simulink model "AttitudeTest"  (R2017b)
settings: Solver=ode45  StartTime=0.0  StopTime=20000  RelTol=1e-6  EnableMultiTasking=on
model workspace: external: MATLAB File C:\Users\Justin\Documents\00 MEng Project\PAN_ADCS\models\AttitudeTest_init.m (data not in the file)
undefined symbols (not defined in the file): accelmax, I, invI, Kd, Kp, muE, q_init, r_FWR, v_FWR, wbn_init, wmax, ww0
libraries: simulink x1
settings Model: Creator=Mason  LastModifiedBy=Justin
settings DataIOCC: LimitDataPoints=on  SaveFormat=Array  SignalLoggingSaveFormat=ModelDataLogs
settings OptimizationCC: ExpressionDepthLimit=2147483647  InitFltsAndDblsToZero=on  LifeSpan=inf
settings DebuggingCC: SaveWithParameterizedLinksMsg=none  UnderspecifiedInitializationDetection=Classic  MergeDetectMultiDrivingBlocksExec=none  SignalResolutionControl=TryResolveAllWithWarning  SolverPrmCheckMsg=warning  MultiTaskDSMMsg=warning  MultiTaskCondExecSysMsg=none  FcnCallInpInsideContextMsg=warning  StateNameClashWarn=warning  SFUnexpectedBacktrackingDiag=warning  SFNoUnconditionalDefaultTransitionDiag=warning  SFExecutionAtInitializationDiag=none
settings HardwareCC: ProdBitPerPointer=32  ProdBitPerSizeT=32  ProdBitPerPtrDiffT=32  ProdLargestAtomicFloat=None  ProdIntDivRoundTo=Undefined  ProdEndianess=Unspecified  ProdWordSize=32  ProdHWDeviceType=32-bit Generic
settings ModelReferenceCC: PropagateSignalLabelsOutOfModel=off
settings CodeAppCC: StateflowObjectComments=on
settings GRTTargetCC: TargetFcnLib=ansi_tfl_tmw.mat  TargetLangStandard=C89/C90 (ANSI)  GeneratePreprocessorConditionals=Disable all  CombineOutputUpdateFcns=off  GRTInterface=on
settings ConfigComp: CovMetricSettings=dw  CovHtmlReporting=on  CovSaveCumulativeToWorkspaceVar=on  CovSaveSingleToWorkspaceVar=on  CovExternalEMLEnable=off

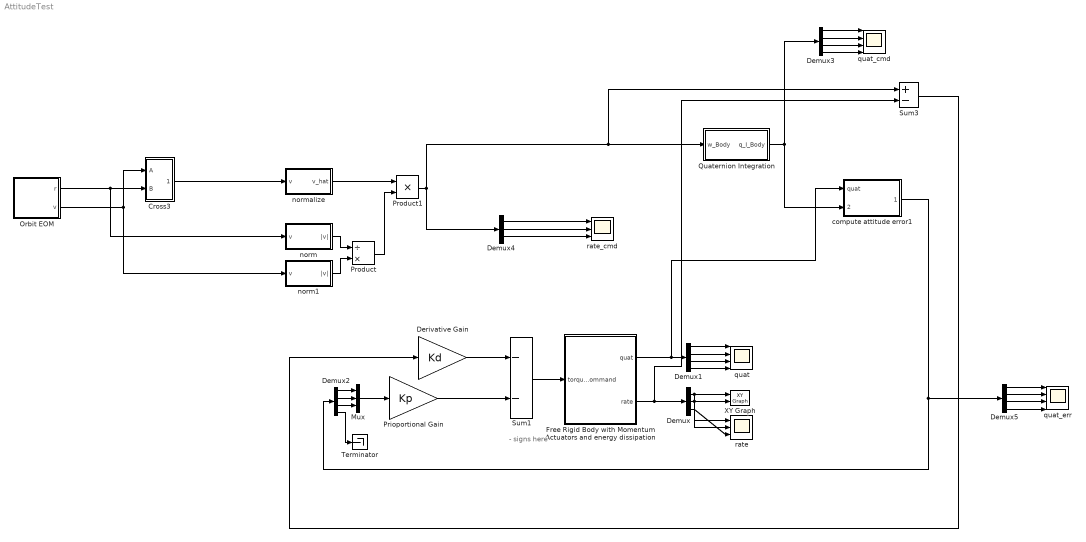
== system AttitudeTest ==
  note: - signs here
  Cross3 : Subsystem
  Demux : Demux  Outputs=3
  Demux{1..3,5} (4 alike) : Demux
  Demux4 : Demux  Outputs=3
  Derivative Gain : Gain  Gain=Kd  SaturateOnIntegerOverflow=on  OutDataTypeStr=Inherit: Same as input  ParamDataTypeStr=Inherit: Same as input
  Free Rigid Body with Momentum Actuators and energy dissipation : Subsystem
  Mux : Mux  Inputs=3
  Orbit EOM : Subsystem
  Prioportional Gain : Gain  Gain=Kp  SaturateOnIntegerOverflow=on  OutDataTypeStr=Inherit: Same as input  ParamDataTypeStr=Inherit: Same as input
  Product : Product  Inputs=/*
  Product1 : Product
  Quaternion Integration : Subsystem
  Sum1 : Sum  Inputs=--  SaturateOnIntegerOverflow=on  InputSameDT=on  OutDataTypeStr=Inherit: Same as first input
  Sum3 : Sum  Inputs=+-  SaturateOnIntegerOverflow=on  InputSameDT=on  OutDataTypeStr=Inherit: Same as first input
  Terminator : Terminator
  XY Graph : simulink/Sinks/XY Graph  xmin=-.1  xmax=.1  ymin=-.1  ymax=.1  st=.25
  compute attitude error1 : Subsystem
  norm : Subsystem
  norm1 : Subsystem
  normalize : Subsystem
  quat : Scope  NumInputPorts=4
  quat_cmd : Scope  NumInputPorts=4
  quat_err : Scope  NumInputPorts=4
  rate : Scope  NumInputPorts=3
  rate_cmd : Scope  NumInputPorts=3
  wires:
  Demux1/1 -> quat/1
  Demux1/2 -> quat/2
  Demux1/3 -> quat/3
  Demux1/4 -> quat/4
  Demux/1 -> rate/1, XY Graph/1
  Demux/2 -> rate/2, XY Graph/2
  Demux/3 -> rate/3
  Free Rigid Body with Momentum Actuators and energy dissipation/2(rate) -> Sum3/2, Demux/1
  Free Rigid Body with Momentum Actuators and energy dissipation/1(quat) -> compute attitude error1/1(quat), Demux1/1
  Sum1/1 -> Free Rigid Body with Momentum Actuators and energy dissipation/1(torque command)
  Mux/1 -> Prioportional Gain/1
  Derivative Gain/1 -> Sum1/1
  Demux2/2 -> Mux/2
  Demux2/1 -> Mux/1
  Demux2/3 -> Mux/3
  Demux2/4 -> Terminator/1
  Prioportional Gain/1 -> Sum1/2
  Quaternion Integration/1(q_I_Body) -> compute attitude error1/2(quat_cmd), Demux3/1
  compute attitude error1/1(quat error) -> Demux5/1, Demux2/1
  Sum3/1 -> Derivative Gain/1
  Product1/1 -> Demux4/1, Sum3/1, Quaternion Integration/1(w_Body)
  Demux3/3 -> quat_cmd/3
  Demux3/2 -> quat_cmd/2
  Demux3/4 -> quat_cmd/4
  Demux3/1 -> quat_cmd/1
  Orbit EOM/1(r) -> norm/1(v), Cross3/2(B)
  normalize/1(v_hat) -> Product1/1
  Product/1 -> Product1/2
  norm/1(|v|) -> Product/1
  Orbit EOM/2(v) -> Cross3/1(A), norm1/1(v)
  Cross3/1(AxB) -> normalize/1(v)
  norm1/1(|v|) -> Product/2
  Demux4/1 -> rate_cmd/1
  Demux4/3 -> rate_cmd/3
  Demux4/2 -> rate_cmd/2
  Demux5/2 -> quat_err/2
  Demux5/1 -> quat_err/1
  Demux5/4 -> quat_err/4
  Demux5/3 -> quat_err/3

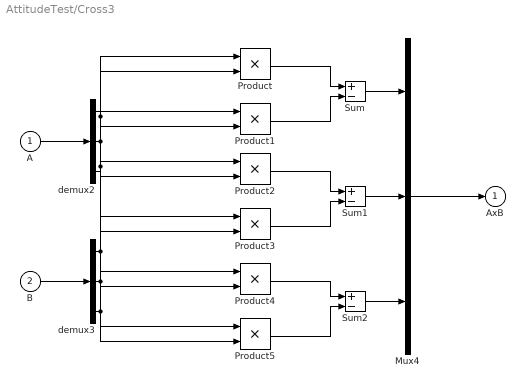
== system AttitudeTest/Cross3 ==
  A : Inport
  B : Inport  Port=2
  Mux4 : Mux  Inputs=3
  Product{,1..5} (6 alike) : Product  SaturateOnIntegerOverflow=on  InputSameDT=on  OutDataTypeStr=Inherit: Same as first input
  Sum : Sum  Inputs=+-  SaturateOnIntegerOverflow=on  InputSameDT=on  OutDataTypeStr=Inherit: Same as first input
  Sum1 : Sum  Inputs=+-  SaturateOnIntegerOverflow=on  InputSameDT=on  OutDataTypeStr=Inherit: Same as first input
  Sum2 : Sum  Inputs=+-  SaturateOnIntegerOverflow=on  InputSameDT=on  OutDataTypeStr=Inherit: Same as first input
  demux2 : Demux  Outputs=3
  demux3 : Demux  Outputs=3
  AxB : Outport  InitialOutput=0
  wires:
  A/1 -> demux2/1
  B/1 -> demux3/1
  demux2/3 -> Product1/1, Product2/1
  demux3/3 -> Product/2, Product3/2
  demux2/1 -> Product3/1, Product4/1
  demux3/2 -> Product1/2, Product4/2
  demux2/2 -> Product/1, Product5/1
  demux3/1 -> Product2/2, Product5/2
  Product/1 -> Sum/1
  Product1/1 -> Sum/2
  Product2/1 -> Sum1/1
  Product3/1 -> Sum1/2
  Product4/1 -> Sum2/1
  Product5/1 -> Sum2/2
  Sum/1 -> Mux4/1
  Sum1/1 -> Mux4/2
  Sum2/1 -> Mux4/3
  Mux4/1 -> AxB/1

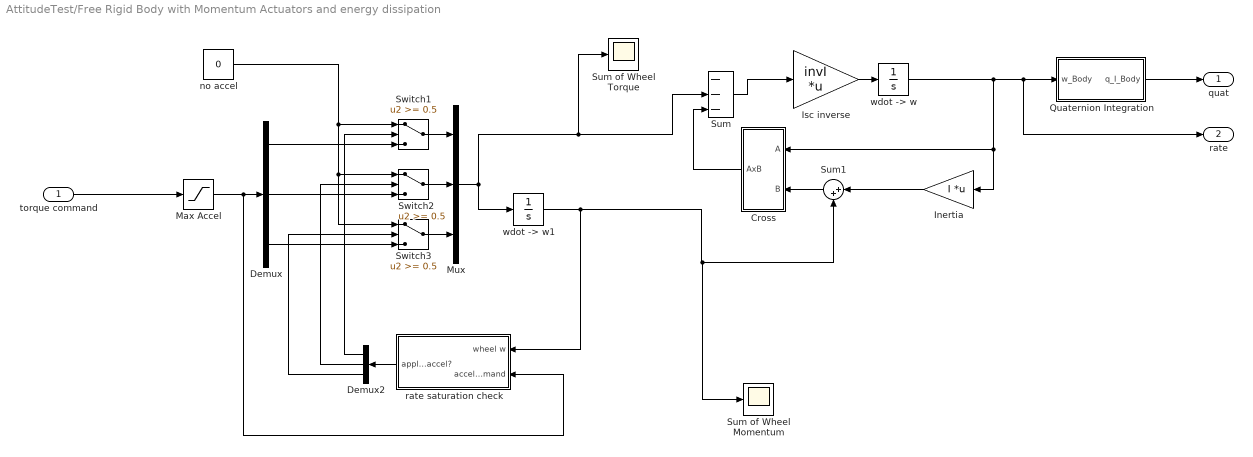
== system AttitudeTest/Free Rigid Body with Momentum Actuators and energy dissipation ==
  torque command : Inport
  Cross : Subsystem
  Demux : Demux  Outputs=3
  Demux2 : Demux  Outputs=3
  Inertia : Gain  Gain=I  Multiplication=Matrix(K*u)  SaturateOnIntegerOverflow=on  OutDataTypeStr=Inherit: Same as input  ParamDataTypeStr=Inherit: Same as input
  Isc inverse : Gain  Gain=invI  Multiplication=Matrix(K*u)  SaturateOnIntegerOverflow=on  OutDataTypeStr=Inherit: Same as input  ParamDataTypeStr=Inherit: Same as input
  Max Accel : Saturate  UpperLimit=accelmax  LowerLimit=-accelmax
  Mux : Mux  Inputs=3
  Quaternion Integration : Subsystem
  Sum : Sum  Inputs=|---  SaturateOnIntegerOverflow=on  InputSameDT=on  OutDataTypeStr=Inherit: Same as first input
  Sum of Wheel Momentum : Scope
  Sum of Wheel Torque : Scope
  Sum1 : Sum  Inputs=|++  SaturateOnIntegerOverflow=on  InputSameDT=on  OutDataTypeStr=Inherit: Same as first input
  Switch1 : Switch  Threshold=0.5  SaturateOnIntegerOverflow=on  InputSameDT=on
  Switch2 : Switch  Threshold=0.5  SaturateOnIntegerOverflow=on  InputSameDT=on
  Switch3 : Switch  Threshold=0.5  SaturateOnIntegerOverflow=on  InputSameDT=on
  no accel : Constant  Value=0
  rate saturation check : Subsystem
  "wdot -> w" : Integrator  InitialCondition=wbn_init
  "wdot -> w1" : Integrator  InitialCondition=ww0
  quat : Outport
  rate : Outport  Port=2
  wires:
  Isc inverse/1 -> "wdot -> w"/1
  "wdot -> w"/1 -> rate/1, Quaternion Integration/1(w_Body), Inertia/1, Cross/1(A)
  Sum/1 -> Isc inverse/1
  Cross/1(AxB) -> Sum/3
  Max Accel/1 -> rate saturation check/2(accel command), Demux/1
  Demux2/1 -> Switch1/2
  Demux2/2 -> Switch2/2
  Demux2/3 -> Switch3/2
  no accel/1 -> Switch1/1, Switch2/1, Switch3/1
  torque command/1 -> Max Accel/1
  Mux/1 -> Sum of Wheel Torque/1, Sum/2, "wdot -> w1"/1
  "wdot -> w1"/1 -> Sum of Wheel Momentum/1, Sum1/2, rate saturation check/1(wheel w)
  Inertia/1 -> Sum1/1
  Sum1/1 -> Cross/2(B)
  Quaternion Integration/1(q_I_Body) -> quat/1
  Switch1/1 -> Mux/1
  Switch2/1 -> Mux/2
  Switch3/1 -> Mux/3
  Demux/1 -> Switch1/3
  Demux/2 -> Switch2/3
  Demux/3 -> Switch3/3
  rate saturation check/1(apply accel?) -> Demux2/1

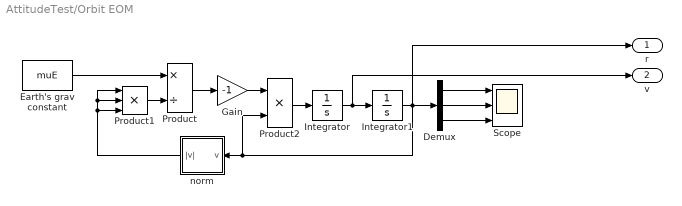
== system AttitudeTest/Orbit EOM ==
  Demux : Demux  Outputs=3
  Earth's grav constant : Constant  Value=muE
  Gain : Gain  Gain=-1  SaturateOnIntegerOverflow=on  OutDataTypeStr=Inherit: Same as input  ParamDataTypeStr=Inherit: Same as input
  Integrator : Integrator  InitialCondition=v_FWR
  Integrator1 : Integrator  InitialCondition=r_FWR
  Product : Product  Inputs=*/  SaturateOnIntegerOverflow=on  OutDataTypeStr=Inherit: Same as first input
  Product1 : Product  Inputs=***  SaturateOnIntegerOverflow=on  OutDataTypeStr=Inherit: Same as first input
  Product2 : Product  Inputs=**  SaturateOnIntegerOverflow=on  OutDataTypeStr=Inherit: Same as first input
  Scope : Scope  NumInputPorts=3
  norm : Subsystem
  r : Outport
  v : Outport  Port=2
  wires:
  norm/1(|v|) -> Product1/3, Product1/2, Product1/1
  Demux/3 -> Scope/3
  Demux/2 -> Scope/2
  Demux/1 -> Scope/1
  Gain/1 -> Product2/1
  Integrator/1 -> v/1, Integrator1/1
  Product2/1 -> Integrator/1
  Product/1 -> Gain/1
  Integrator1/1 -> r/1, Demux/1, norm/1(v), Product2/2
  Product1/1 -> Product/2
  Earth's grav constant/1 -> Product/1

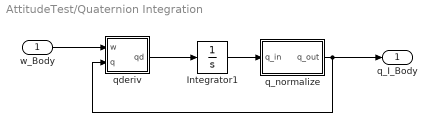
== system AttitudeTest/Quaternion Integration ==
  w_Body : Inport
  Integrator1 : Integrator  InitialCondition=q_init
  q_normalize : Subsystem
  qderiv : Subsystem
  q_I_Body : Outport
  wires:
  w_Body/1 -> qderiv/1(w)
  q_normalize/1(q_out) -> qderiv/2(q), q_I_Body/1
  Integrator1/1 -> q_normalize/1(q_in)
  qderiv/1(qd) -> Integrator1/1

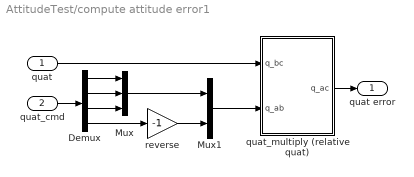
== system AttitudeTest/compute attitude error1 ==
  quat : Inport
  quat_cmd : Inport  Port=2
  Demux : Demux
  Mux : Mux  Inputs=3
  Mux1 : Mux  Inputs=2
  quat_multiply (relative quat) : Subsystem
  reverse : Gain  Gain=-1  SaturateOnIntegerOverflow=on  OutDataTypeStr=Inherit: Same as input  ParamDataTypeStr=Inherit: Same as input
  quat error : Outport
  wires:
  quat/1 -> quat_multiply (relative quat)/1(q_bc)
  quat_cmd/1 -> Demux/1
  Demux/1 -> Mux/1
  Demux/2 -> Mux/2
  Demux/3 -> Mux/3
  Demux/4 -> reverse/1
  Mux/1 -> Mux1/1
  Mux1/1 -> quat_multiply (relative quat)/2(q_ab)
  reverse/1 -> Mux1/2
  quat_multiply (relative quat)/1(q_ac) -> quat error/1

== system AttitudeTest/norm ==
  v : Inport
  Dot Product : DotProduct  InputSameDT=on  OutDataTypeStr=Inherit: Inherit via internal rule
  Math Function : Math  Operator=sqrt  SaturateOnIntegerOverflow=on
  |v| : Outport
  wires:
  Math Function/1 -> |v|/1
  Dot Product/1 -> Math Function/1
  v/1 -> Dot Product/2, Dot Product/1

== system AttitudeTest/norm1 ==
  v : Inport
  Dot Product : DotProduct  InputSameDT=on  OutDataTypeStr=Inherit: Inherit via internal rule
  Math Function : Math  Operator=sqrt  SaturateOnIntegerOverflow=on
  |v| : Outport
  wires:
  v/1 -> Dot Product/1, Dot Product/2
  Dot Product/1 -> Math Function/1
  Math Function/1 -> |v|/1

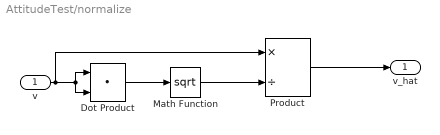
== system AttitudeTest/normalize ==
  v : Inport
  Dot Product : DotProduct  InputSameDT=on  OutDataTypeStr=Inherit: Inherit via internal rule
  Math Function : Math  Operator=sqrt  SaturateOnIntegerOverflow=on
  Product : Product  Inputs=*/  SaturateOnIntegerOverflow=on  InputSameDT=on  OutDataTypeStr=Inherit: Same as first input
  v_hat : Outport
  wires:
  v/1 -> Dot Product/1, Dot Product/2, Product/1
  Dot Product/1 -> Math Function/1
  Math Function/1 -> Product/2
  Product/1 -> v_hat/1

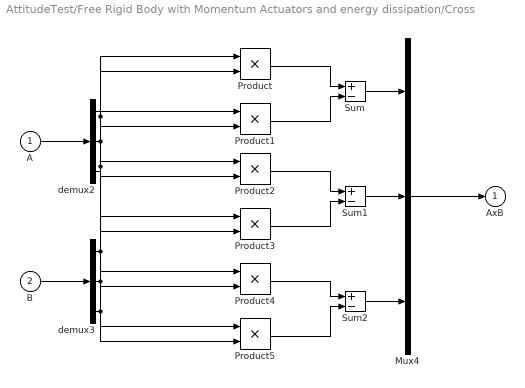
== system AttitudeTest/Free Rigid Body with Momentum Actuators and energy dissipation/Cross ==
  A : Inport
  B : Inport  Port=2
  Mux4 : Mux  Inputs=3
  Product{,1..5} (6 alike) : Product  SaturateOnIntegerOverflow=on  InputSameDT=on  OutDataTypeStr=Inherit: Same as first input
  Sum : Sum  Inputs=+-  SaturateOnIntegerOverflow=on  InputSameDT=on  OutDataTypeStr=Inherit: Same as first input
  Sum1 : Sum  Inputs=+-  SaturateOnIntegerOverflow=on  InputSameDT=on  OutDataTypeStr=Inherit: Same as first input
  Sum2 : Sum  Inputs=+-  SaturateOnIntegerOverflow=on  InputSameDT=on  OutDataTypeStr=Inherit: Same as first input
  demux2 : Demux  Outputs=3
  demux3 : Demux  Outputs=3
  AxB : Outport  InitialOutput=0
  wires:
  A/1 -> demux2/1
  B/1 -> demux3/1
  demux2/3 -> Product1/1, Product2/1
  demux3/3 -> Product/2, Product3/2
  demux2/1 -> Product3/1, Product4/1
  demux3/2 -> Product1/2, Product4/2
  demux2/2 -> Product/1, Product5/1
  demux3/1 -> Product2/2, Product5/2
  Product/1 -> Sum/1
  Product1/1 -> Sum/2
  Product2/1 -> Sum1/1
  Product3/1 -> Sum1/2
  Product4/1 -> Sum2/1
  Product5/1 -> Sum2/2
  Sum/1 -> Mux4/1
  Sum1/1 -> Mux4/2
  Sum2/1 -> Mux4/3
  Mux4/1 -> AxB/1

== system AttitudeTest/Free Rigid Body with Momentum Actuators and energy dissipation/Quaternion Integration ==
  w_Body : Inport
  Integrator1 : Integrator  InitialCondition=q_init
  q_normalize : Subsystem
  qderiv : Subsystem
  q_I_Body : Outport
  wires:
  w_Body/1 -> qderiv/1(w)
  q_normalize/1(q_out) -> qderiv/2(q), q_I_Body/1
  Integrator1/1 -> q_normalize/1(q_in)
  qderiv/1(qd) -> Integrator1/1

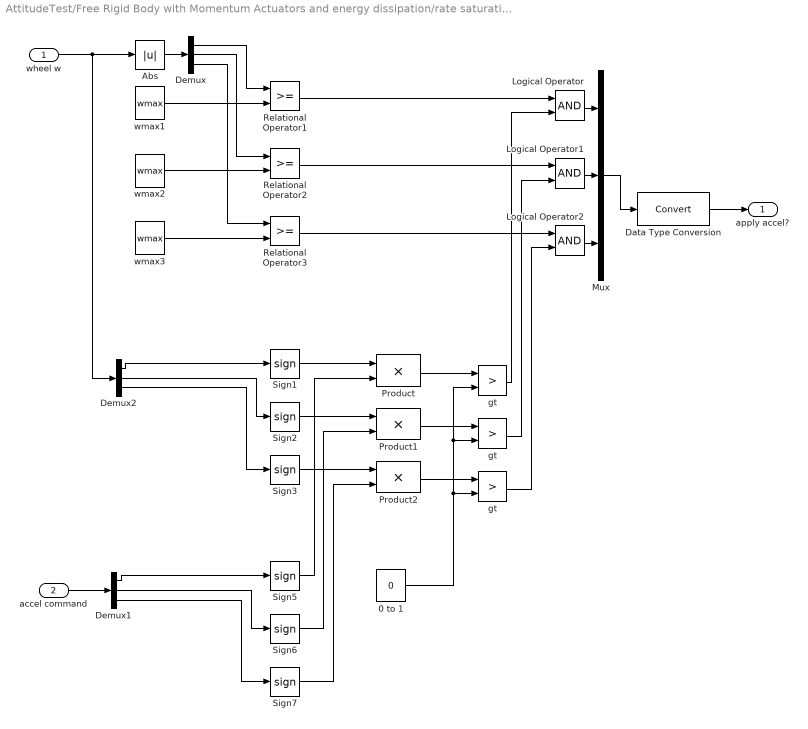
== system AttitudeTest/Free Rigid Body with Momentum Actuators and energy dissipation/rate saturation check ==
  wheel w : Inport
  accel command : Inport  Port=2
  0 to 1 : Constant  Value=0  VectorParams1D=off
  Abs : Abs  SaturateOnIntegerOverflow=on
  Data Type Conversion : DataTypeConversion
  Demux : Demux  Outputs=3
  Demux1 : Demux  Outputs=3
  Demux2 : Demux  Outputs=3
  Logical Operator : Logic
  Logical Operator1 : Logic
  Logical Operator2 : Logic
  Mux : Mux  Inputs=3
  Product : Product  SaturateOnIntegerOverflow=on  InputSameDT=on  OutDataTypeStr=Inherit: Same as first input
  Product1 : Product  SaturateOnIntegerOverflow=on  InputSameDT=on  OutDataTypeStr=Inherit: Same as first input
  Product2 : Product  SaturateOnIntegerOverflow=on  InputSameDT=on  OutDataTypeStr=Inherit: Same as first input
  Relational Operator1 : RelationalOperator  RndMeth=Nearest  InputSameDT=on
  Relational Operator2 : RelationalOperator  RndMeth=Nearest  InputSameDT=on
  Relational Operator3 : RelationalOperator  RndMeth=Nearest  InputSameDT=on
  Sign{1..3,5..7} (6 alike) : Signum
  gt : RelationalOperator  Operator=>  RndMeth=Nearest  InputSameDT=on
  "gt " : RelationalOperator  Operator=>  RndMeth=Nearest  InputSameDT=on
  "gt  " : RelationalOperator  Operator=>  RndMeth=Nearest  InputSameDT=on
  wmax1 : Constant  Value=wmax  VectorParams1D=off
  wmax2 : Constant  Value=wmax  VectorParams1D=off
  wmax3 : Constant  Value=wmax  VectorParams1D=off
  apply accel? : Outport
  wires:
  Abs/1 -> Demux/1
  Demux/1 -> Relational Operator1/1
  Demux/2 -> Relational Operator2/1
  Demux/3 -> Relational Operator3/1
  wmax1/1 -> Relational Operator1/2
  wmax2/1 -> Relational Operator2/2
  wmax3/1 -> Relational Operator3/2
  wheel w/1 -> Abs/1, Demux2/1
  Mux/1 -> Data Type Conversion/1
  accel command/1 -> Demux1/1
  Demux1/2 -> Sign6/1
  Demux1/3 -> Sign7/1
  Sign1/1 -> Product/1
  Sign5/1 -> Product/2
  Sign2/1 -> Product1/1
  Sign6/1 -> Product1/2
  Sign3/1 -> Product2/1
  Sign7/1 -> Product2/2
  Product/1 -> gt/1
  Product1/1 -> "gt "/1
  Product2/1 -> "gt  "/1
  Logical Operator/1 -> Mux/1
  Logical Operator1/1 -> Mux/2
  Logical Operator2/1 -> Mux/3
  Relational Operator1/1 -> Logical Operator/1
  Relational Operator2/1 -> Logical Operator1/1
  Relational Operator3/1 -> Logical Operator2/1
  gt/1 -> Logical Operator/2
  "gt "/1 -> Logical Operator1/2
  "gt  "/1 -> Logical Operator2/2
  Demux2/1 -> Sign1/1
  Demux2/2 -> Sign2/1
  Demux2/3 -> Sign3/1
  0 to 1/1 -> "gt  "/2, "gt "/2, gt/2
  Demux1/1 -> Sign5/1
  Data Type Conversion/1 -> apply accel?/1

== system AttitudeTest/Orbit EOM/norm ==
  v : Inport
  Dot Product : DotProduct  InputSameDT=on  OutDataTypeStr=Inherit: Inherit via internal rule
  Math Function : Math  Operator=sqrt  SaturateOnIntegerOverflow=on
  Saturation : Saturate  UpperLimit=1e20  LowerLimit=1e-10
  |v| : Outport
  wires:
  Saturation/1 -> |v|/1
  Math Function/1 -> Saturation/1
  Dot Product/1 -> Math Function/1
  v/1 -> Dot Product/2, Dot Product/1

== system AttitudeTest/Quaternion Integration/q_normalize ==
  q_in : Inport  PortDimensions=4
  Dot Product : DotProduct  InputSameDT=on  OutDataTypeStr=Inherit: Inherit via internal rule
  Math Function : Math  Operator=sqrt  SaturateOnIntegerOverflow=on
  Product : Product  Inputs=*/  SaturateOnIntegerOverflow=on  InputSameDT=on  OutDataTypeStr=Inherit: Same as first input
  q_out : Outport
  wires:
  Product/1 -> q_out/1
  Math Function/1 -> Product/2
  Dot Product/1 -> Math Function/1
  q_in/1 -> Product/1, Dot Product/2, Dot Product/1

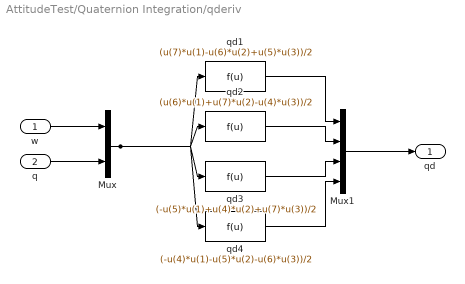
== system AttitudeTest/Quaternion Integration/qderiv ==
  w : Inport
  q : Inport  Port=2
  Mux : Mux  Inputs=2
  Mux1 : Mux
  qd1 : Fcn  Expr=(u(7)*u(1)-u(6)*u(2)+u(5)*u(3))/2
  qd2 : Fcn  Expr=(u(6)*u(1)+u(7)*u(2)-u(4)*u(3))/2
  qd3 : Fcn  Expr=(-u(5)*u(1)+u(4)*u(2)+u(7)*u(3))/2
  qd4 : Fcn  Expr=(-u(4)*u(1)-u(5)*u(2)-u(6)*u(3))/2
  qd : Outport
  wires:
  Mux1/1 -> qd/1
  qd4/1 -> Mux1/4
  qd3/1 -> Mux1/3
  qd2/1 -> Mux1/2
  qd1/1 -> Mux1/1
  Mux/1 -> qd4/1, qd3/1, qd2/1, qd1/1
  q/1 -> Mux/2
  w/1 -> Mux/1

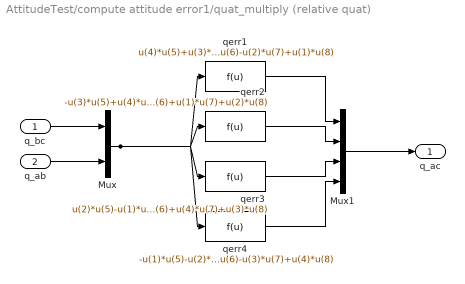
== system AttitudeTest/compute attitude error1/quat_multiply (relative quat) ==
  q_bc : Inport
  q_ab : Inport  Port=2
  Mux : Mux  Inputs=2
  Mux1 : Mux
  qerr1 : Fcn  Expr=u(4)*u(5)+u(3)*u(6)-u(2)*u(7)+u(1)*u(8)
  qerr2 : Fcn  Expr=-u(3)*u(5)+u(4)*u(6)+u(1)*u(7)+u(2)*u(8)
  qerr3 : Fcn  Expr=u(2)*u(5)-u(1)*u(6)+u(4)*u(7)+u(3)*u(8)
  qerr4 : Fcn  Expr=-u(1)*u(5)-u(2)*u(6)-u(3)*u(7)+u(4)*u(8)
  q_ac : Outport
  wires:
  Mux1/1 -> q_ac/1
  qerr4/1 -> Mux1/4
  qerr3/1 -> Mux1/3
  qerr2/1 -> Mux1/2
  qerr1/1 -> Mux1/1
  Mux/1 -> qerr4/1, qerr3/1, qerr2/1, qerr1/1
  q_ab/1 -> Mux/2
  q_bc/1 -> Mux/1

== system AttitudeTest/Free Rigid Body with Momentum Actuators and energy dissipation/Quaternion Integration/q_normalize ==
  q_in : Inport  PortDimensions=4
  Dot Product : DotProduct  InputSameDT=on  OutDataTypeStr=Inherit: Inherit via internal rule
  Math Function : Math  Operator=sqrt  SaturateOnIntegerOverflow=on
  Product : Product  Inputs=*/  SaturateOnIntegerOverflow=on  InputSameDT=on  OutDataTypeStr=Inherit: Same as first input
  q_out : Outport
  wires:
  Product/1 -> q_out/1
  Math Function/1 -> Product/2
  Dot Product/1 -> Math Function/1
  q_in/1 -> Product/1, Dot Product/2, Dot Product/1

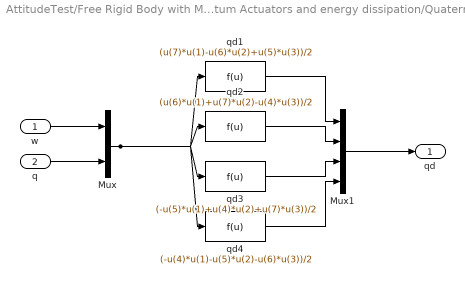
== system AttitudeTest/Free Rigid Body with Momentum Actuators and energy dissipation/Quaternion Integration/qderiv ==
  w : Inport
  q : Inport  Port=2
  Mux : Mux  Inputs=2
  Mux1 : Mux
  qd1 : Fcn  Expr=(u(7)*u(1)-u(6)*u(2)+u(5)*u(3))/2
  qd2 : Fcn  Expr=(u(6)*u(1)+u(7)*u(2)-u(4)*u(3))/2
  qd3 : Fcn  Expr=(-u(5)*u(1)+u(4)*u(2)+u(7)*u(3))/2
  qd4 : Fcn  Expr=(-u(4)*u(1)-u(5)*u(2)-u(6)*u(3))/2
  qd : Outport
  wires:
  Mux1/1 -> qd/1
  qd4/1 -> Mux1/4
  qd3/1 -> Mux1/3
  qd2/1 -> Mux1/2
  qd1/1 -> Mux1/1
  Mux/1 -> qd4/1, qd3/1, qd2/1, qd1/1
  q/1 -> Mux/2
  w/1 -> Mux/1
